simulink model "P1"  (R2025a)
settings: Solver=ode45  StartTime=0.0  StopTime=500  RelTol=1e-3
values from neighbouring files (symbols this model uses):
  Beq = 4.3    [P1.m]
  Bp = 0.0024    [P1.m]
  Fc = 0    [P1.m]
  g = 9.81    [P1.m]
  Ip = 0.0079    [P1.m]
  lp = 0.3302    [P1.m]
  Mc = 0.7031    [P1.m]
  Mp = 0.23    [P1.m]
settings Model: LastModifiedBy=ernes

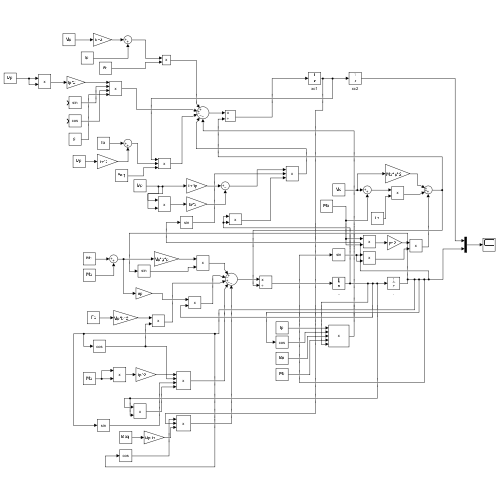
[thumbnail: Simulink's stored preview of the top-level diagram]
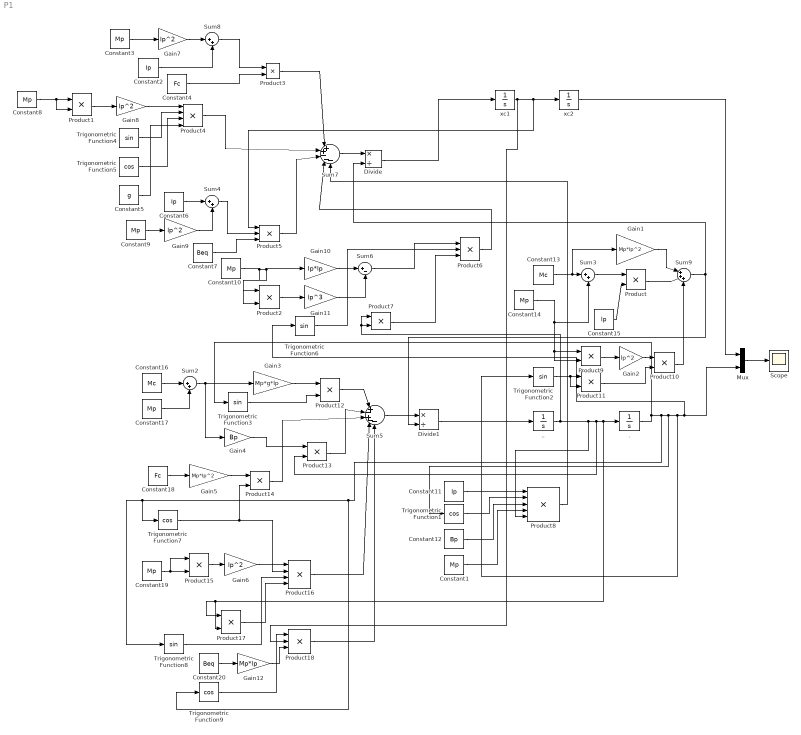
== system P1 ==
  . : Integrator  InitialCondition=0.01745
  .. : Integrator
  Constant{1,3,8..10,14,17,19} (8 alike) : Constant  Value=Mp
  Constant11 : Constant  Value=lp
  Constant12 : Constant  Value=Bp
  Constant13 : Constant  Value=Mc
  Constant15 : Constant  Value=lp
  Constant16 : Constant  Value=Mc
  Constant18 : Constant  Value=Fc
  Constant2 : Constant  Value=Ip
  Constant20 : Constant  Value=Beq
  Constant4 : Constant  Value=Fc
  Constant5 : Constant  Value=g
  Constant6 : Constant  Value=Ip
  Constant7 : Constant  Value=Beq
  Divide : Product  Inputs=*/
  Divide1 : Product  Inputs=*/
  Gain1 : Gain  Gain=Mp*lp^2
  Gain10 : Gain  Gain=Ip*lp
  Gain11 : Gain  Gain=lp^3
  Gain12 : Gain  Gain=Mp*lp
  Gain{2,6..9} (5 alike) : Gain  Gain=lp^2
  Gain3 : Gain  Gain=Mp*g*lp
  Gain4 : Gain  Gain=Bp
  Gain5 : Gain  Gain=Mp*lp^2
  Mux : Mux  Inputs=2
  Product{,1..3,7,9..15,17} (13 alike) : Product
  Product16 : Product  Inputs=4
  Product18 : Product  Inputs=3
  Product4 : Product  Inputs=4
  Product5 : Product  Inputs=3
  Product6 : Product  Inputs=3
  Product8 : Product  Inputs=5
  Scope : Scope
      settings: ActiveDisplayYMinimum=-6.0786230445401523  ActiveDisplayYMaximum=9.5925870432442775
  Sum{2..4,8} (4 alike) : Sum  Inputs=|++
  Sum5 : Sum  Inputs=|+-+--
  Sum6 : Sum  Inputs=|+-
  Sum7 : Sum  Inputs=|++---
  Sum9 : Sum  Inputs=|+++
  Trigonometric Function{1,5,7,9} (4 alike) : Trigonometry  Operator=cos
  Trigonometric Function{2..4,6,8} (5 alike) : Trigonometry
  xc1 : Integrator
  xc2 : Integrator
  wires:
  Constant3/1 -> Gain7/1
  Gain7/1 -> Sum8/1
  Constant2/1 -> Sum8/2
  Sum8/1 -> Product3/1
  Constant4/1 -> Product3/2
  Product3/1 -> Sum7/1
  Gain8/1 -> Product4/1
  Constant5/1 -> Product4/4
  Trigonometric Function4/1 -> Product4/2
  Trigonometric Function5/1 -> Product4/3
  Product4/1 -> Sum7/2
  Constant6/1 -> Sum4/1
  Gain9/1 -> Sum4/2
  Sum4/1 -> Product5/2
  Constant7/1 -> Product5/3
  Divide/1 -> xc1/1
  Product5/1 -> Sum7/3
  Gain10/1 -> Sum6/1
  Gain11/1 -> Sum6/2
  Sum6/1 -> Product6/1
  Product7/1 -> Product6/3
  Trigonometric Function6/1 -> Product6/2
  Constant8/1 -> Product1/2, Product1/1
  Constant9/1 -> Gain9/1
  Constant10/1 -> Product2/2, Gain10/1, Product2/1
  Product2/1 -> Gain11/1
  Product6/1 -> Sum7/4
  Constant1/1 -> Product8/4
  Constant11/1 -> Product8/1
  Trigonometric Function1/1 -> Product8/2
  Constant12/1 -> Product8/3
  Product8/1 -> Sum7/5
  Constant13/1 -> Gain1/1, Sum3/1
  Constant14/1 -> Product9/2, Product9/1, Sum3/2
  Constant15/1 -> Product/2
  Sum3/1 -> Product/1
  Gain1/1 -> Sum9/1
  Product/1 -> Sum9/2
  Trigonometric Function2/1 -> Product11/2, Product11/1
  Product11/1 -> Product10/2
  Product10/1 -> Sum9/3
  Constant16/1 -> Sum2/1
  Constant17/1 -> Sum2/2
  Sum2/1 -> Gain4/1, Gain3/1
  Gain3/1 -> Product12/1
  Trigonometric Function3/1 -> Product12/2
  Product12/1 -> Sum5/1
  Gain4/1 -> Product13/1
  Product13/1 -> Sum5/2
  Constant18/1 -> Gain5/1
  Gain5/1 -> Product14/1
  Trigonometric Function7/1 -> Product16/2, Product14/2
  Product14/1 -> Sum5/3
  Constant19/1 -> Product15/2, Product15/1
  Gain6/1 -> Product16/1
  Product17/1 -> Product16/4
  ../1 -> Product8/5, ./1, Product17/2, Product17/1, Product13/2, Product7/1, Product7/2
  Trigonometric Function8/1 -> Product16/3
  Product16/1 -> Sum5/4
  Constant20/1 -> Gain12/1
  Gain12/1 -> Product18/3
  xc1/1 -> Product5/1, xc2/1, Product18/2
  Trigonometric Function9/1 -> Product18/1
  Product18/1 -> Sum5/5
  Sum5/1 -> Divide1/1
  Sum9/1 -> Divide/2, Divide1/2
  xc2/1 -> Mux/1
  Divide1/1 -> ../1
  Mux/1 -> Scope/1
  ./1 -> Trigonometric Function9/1, Trigonometric Function8/1, Trigonometric Function7/1, Trigonometric Function1/1, Mux/2, Trigonometric Function6/1, Trigonometric Function2/1, Trigonometric Function3/1
  Sum7/1 -> Divide/1
  Product1/1 -> Gain8/1
  Product9/1 -> Gain2/1
  Gain2/1 -> Product10/1
  Product15/1 -> Gain6/1
